simulink model "test"  (Simulink 6.4)
settings: Solver=FixedStepDiscrete  StartTime=0.0  StopTime=10.0  FixedStep=1  RelTol=1e-3
libraries: simulink x2
settings Model: Creator=brownm5  LastModifiedBy=brownm5
settings OptimizationCC: InlineInvariantSignals=on
settings DebuggingCC: StrictBusMsg=None
settings HardwareCC: TargetHWDeviceType=32-bit Generic

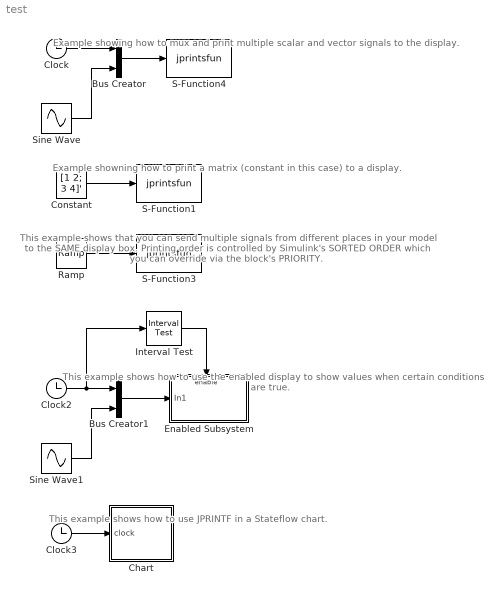
== system test ==
  note: Example showing how to mux and print multiple
      | scalar and vector signals to the display.
  note: Example showning how to print a matrix (constant
      | in this case) to a display.
  note: This example shows that you can send multiple
      | signals from different places in your model to
      | the SAME display box.  Printing order is controlled
      | by Simulink's SORTED ORDER which you can
      | override via the block's PRIORITY.
  note: This example shows how to use the enabled
      | display to show values when certain
      | conditions are true.
  note: This example shows how to use JPRINTF in a Stateflow chart.
  Bus Creator : BusCreator  Inputs=2
  Bus Creator1 : BusCreator  Inputs=2
  Chart : Stateflow chart  TreatAsAtomicUnit=on
      settings: PermitHierarchicalResolution=ParametersOnly
  Clock : Clock
      settings: Decimation=10
  Clock2 : Clock
      settings: Decimation=10
  Clock3 : Clock
      settings: Decimation=10
  Constant : Constant  Value=[1 2; 3 4]'  OutDataType=sfix(16)  OutScaling=2^0  SampleTime=1
  Enabled Subsystem : Subsystem  TreatAsAtomicUnit=on  mask(Java Display Box){dev=2, fmt1=Time\t\tSine 1\t\tSine 2\n, fmt2=, fmt3=%4.1f\t\t%6.3f\t\t%6.3f, fmt4=\n, fmt5=\nFinal values:\n, fmt6=%4.1f\t\t%6.3f\t\t%6.3f, fmt7=\n\n}
      mask prompts: dev "Display number"; fmt1 "Initialization format"; fmt2 "Update leader format"; fmt3 "Update numeric format"; fmt4 "Update trailer format"; fmt5 "Termination leader format"; fmt6 "Termination numeric format"; fmt7 "Termination trailer format"
      mask help:
      | Displays formatted text and numeric data to an editable Java window.
      | "Display Number" is a positive integer which specifies the Java window to receive the formatted output. Seven format strings control the appearance of the output during block initialization, update, and termination.  These strings can contain any combination of text and format specifiers acceptable to the Matlab FPRINTF function.
      |
      | See HELP for more information.
      mask Help:
      | <HTML>
      | 
      | <head>
      | <TITLE>Java Display Box</TITLE>
      | </head>
      | 
      | <body>
      | 
      | <h2>Function</h2>
      | Displays formatted text and numeric data to an editable Java window.
      | "Display Number" is a positive integer which specifies the Java window to receive the
      | formatted output. Seven format strings control the appearance of the output during
      | block initialization, update, and termination.  These strings can contain any combination
      | of text and format specifiers acceptable to the Matlab FPRINTF function.
      | 
      | <h2>Inputs</h2>
      | Java Display Box accepts any Simulink scalar, vector, or matrix signal.  The signal
      | must be real and double precision.  It is up to the user to perform data type conversion
      | (e.g. int8 to double) and to break apart complex signals into separate real and
      | imaginary parts.  This function will accept multiplexed signals and bus signals.  When
      | displaying matrix signals, Java Display Box will access the matrix data in columnwise
      | order, so you may need to transpose the matrix to display the matrix in it's natural
      | orientation.
      | 
      | <h2>Parameters</h2>
      | 
      | <h3>Display Number:</h3>
      | The display number is a numeric identifier for each active Java Display Box.  Any
      | positive integer greater than zero is acceptable.  If you want the outputs to go do
      | different windows, use differerent Display Numbers for each Java Display Box.
      | You can send multiple signals to the same window by using the same Display
      | Number.  In this case, the order in which the output is written to the box depends on
      | Simulink's execution order, called Sorted Order.  You can force multiple outputs to be
      | displayed in any desired sequence by overriding Simulink's Sorted Order using the
      | block priority property.  To change a Java Display Box priority, right-click the Java Box,
      | select Block  Properties, and enter a numeric value for Block Priority.  The lower the
      | number, the higher the priority, so a good rule of thumb is to assign priorities in the
      | order in which  you want the output to appear in the Java Display Box.
      | <br><br>
      | Note that multiple models share the same set of Java Display Boxes, so if you have
      | more than one model open and those models all access Display Box 1, then the
      | outputs from both models will appear in the same display window.
      | <br><br>
      | If you set the Display Number to -1, the outputs will go to the "standard output", normally
      | the Matlab command window.  A Display Number of -2 will send output to "standard
      | error", and a Display Number consisting of a valid handle to an open file will cause
      | the output to be written to the file.  The user is responsible for opening and closing
      | the file, and passing the file handle to Java Display Box.
      | 
      | <h3>Initialization Format:</h3>
      | The initialization format string is written once during model initialization.  Enter any valid
      | format string (without quotation marks!).  Note that during initialization, the input signal
      | values are generally undefined, so it is not possible to display numeric values of input
      | signals during initialization.  The Initialization Format is generally useful for printing
      | column headers or other delimiters to mark the beginning of a simulation run.  If you
      | don't want any initialization format, leave this field completely blank (i.e. no spaces or
      | other characters).
      | 
      | <h3>Update Format:</h3>
      | The update format strings consist of three parts:  Leader Format, Numeric Format, and
      | Trailer Format.  At each Simulink update time step, the Leader Format is first written
      | once.  Then the Numeric Format is applied to the input signal data, and repeated as
      | necessary to display all of the inputs.  Finally, the Trailer Format is written.  Typically,
      | the Leader Format contains textual information, such as 'Signal Amplitude = ', the
      | Numeric Format contains number formatting strings such as '%6.4f', and the Trailer
      | Format contains units and carriage controls such as '(volts)\n'.
      | 
      | <br><br>Be carefull!  If you have a lengthy simulation, or one that involves many time
      | steps, you can overrun the display memory.  If this is a possibility, consider using a
      | downsampler block in front of the Java Display Box, or enclose it in a triggered
      | subsystem so that only selected time samples are displayed.  If you don't want a
      | Leader, Numeric, or Trailer format, leave the field completely blank.
      | 
      | <h3>Termination Format:</h3>
      | The termination format string consists of three parts:  Leader Format, Numeric Format,
      | and Trailer Format.   These three formats are applied once at the end of a Simulink
      | simulation run.   First, the Leader Format is written once.  Then the Numeric Format is
      | applied to the input signal data, and repeated as necessary to display all of the inputs.
      | Finally, the Trailer Format is written.  Typically, the Leader Format contains textual
      | information, such as 'Signal Amplitude = ', the Numeric Format contains number
      | formatting strings such as '%6.4f', and the Trailer Format contains units and carriage
      | controls such as '(volts)\n'.  These formats are useful if you only want to display the
      | final values of signals at the end of simulation.  You can also use these fields to print
      | summary information, or model termination status.  If you don't want a Leader,
      | Numeric, or Trailer format, leave the field completely blank.
      | 
      | <h2>Java Display Box Menu:</h2>
      | These are fairly self-explanatory.  See HELP on the Java Box pulldown menu for more information.
      | 
      | </body>
      | 
      | </html>
      mask Display: fprintf('Enabled\nJava Box %d',dev)
  Interval Test : simulink/Logic and Bit Operations/Interval Test  SystemSampleTime=-1  IntervalClosedRight=on  uplimit=8  IntervalClosedLeft=on  lowlimit=5  LogicOutDataTypeMode=boolean
  Ramp : simulink/Sources/Ramp  SystemSampleTime=-1  slope=pi  start=0  X0=0
  S-Function1 : S-Function  Priority=4  FunctionName=jprintsfun  Parameters=dev,{fmt1,fmt2,fmt3,fmt4,fmt5,fmt6,fmt7}  EnableBusSupport=off  mask(Java Display Box){dev=1, fmt1=, fmt2=Matrix:\n, fmt3=\t%g\t%g\n, fmt4=\n, fmt5=, fmt6=, fmt7=}
      mask prompts: dev "Display number"; fmt1 "Initialization format"; fmt2 "Update leader format"; fmt3 "Update numeric format"; fmt4 "Update trailer format"; fmt5 "Termination leader format"; fmt6 "Termination numeric format"; fmt7 "Termination trailer format"
      mask help:
      | Displays formatted text and numeric data to an editable Java window.
      | "Display Number" is a positive integer which specifies the Java window to receive the formatted output. Seven format strings control the appearance of the output during block initialization, update, and termination.  These strings can contain any combination of text and format specifiers acceptable to the Matlab FPRINTF function.
      |
      | See HELP for more information.
      mask Help:
      | <HTML>
      | 
      | <head>
      | <TITLE>Java Display Box</TITLE>
      | </head>
      | 
      | <body>
      | 
      | <h2>Function</h2>
      | Displays formatted text and numeric data to an editable Java window.
      | "Display Number" is a positive integer which specifies the Java window to receive the
      | formatted output. Seven format strings control the appearance of the output during
      | block initialization, update, and termination.  These strings can contain any combination
      | of text and format specifiers acceptable to the Matlab FPRINTF function.
      | 
      | <h2>Inputs</h2>
      | Java Display Box accepts any Simulink scalar, vector, or matrix signal.  The signal
      | must be real and double precision.  It is up to the user to perform data type conversion
      | (e.g. int8 to double) and to break apart complex signals into separate real and
      | imaginary parts.  This function will accept multiplexed signals and bus signals.  When
      | displaying matrix signals, Java Display Box will access the matrix data in columnwise
      | order, so you may need to transpose the matrix to display the matrix in it's natural
      | orientation.
      | 
      | <h2>Parameters</h2>
      | 
      | <h3>Display Number:</h3>
      | The display number is a numeric identifier for each active Java Display Box.  Any
      | positive integer greater than zero is acceptable.  If you want the outputs to go do
      | different windows, use differerent Display Numbers for each Java Display Box.
      | You can send multiple signals to the same window by using the same Display
      | Number.  In this case, the order in which the output is written to the box depends on
      | Simulink's execution order, called Sorted Order.  You can force multiple outputs to be
      | displayed in any desired sequence by overriding Simulink's Sorted Order using the
      | block priority property.  To change a Java Display Box priority, right-click the Java Box,
      | select Block  Properties, and enter a numeric value for Block Priority.  The lower the
      | number, the higher the priority, so a good rule of thumb is to assign priorities in the
      | order in which  you want the output to appear in the Java Display Box.
      | <br><br>
      | Note that multiple models share the same set of Java Display Boxes, so if you have
      | more than one model open and those models all access Display Box 1, then the
      | outputs from both models will appear in the same display window.
      | <br><br>
      | If you set the Display Number to -1, the outputs will go to the "standard output", normally
      | the Matlab command window.  A Display Number of -2 will send output to "standard
      | error", and a Display Number consisting of a valid handle to an open file will cause
      | the output to be written to the file.  The user is responsible for opening and closing
      | the file, and passing the file handle to Java Display Box.
      | 
      | <h3>Initialization Format:</h3>
      | The initialization format string is written once during model initialization.  Enter any valid
      | format string (without quotation marks!).  Note that during initialization, the input signal
      | values are generally undefined, so it is not possible to display numeric values of input
      | signals during initialization.  The Initialization Format is generally useful for printing
      | column headers or other delimiters to mark the beginning of a simulation run.  If you
      | don't want any initialization format, leave this field completely blank (i.e. no spaces or
      | other characters).
      | 
      | <h3>Update Format:</h3>
      | The update format strings consist of three parts:  Leader Format, Numeric Format, and
      | Trailer Format.  At each Simulink update time step, the Leader Format is first written
      | once.  Then the Numeric Format is applied to the input signal data, and repeated as
      | necessary to display all of the inputs.  Finally, the Trailer Format is written.  Typically,
      | the Leader Format contains textual information, such as 'Signal Amplitude = ', the
      | Numeric Format contains number formatting strings such as '%6.4f', and the Trailer
      | Format contains units and carriage controls such as '(volts)\n'.
      | 
      | <br><br>Be carefull!  If you have a lengthy simulation, or one that involves many time
      | steps, you can overrun the display memory.  If this is a possibility, consider using a
      | downsampler block in front of the Java Display Box, or enclose it in a triggered
      | subsystem so that only selected time samples are displayed.  If you don't want a
      | Leader, Numeric, or Trailer format, leave the field completely blank.
      | 
      | <h3>Termination Format:</h3>
      | The termination format string consists of three parts:  Leader Format, Numeric Format,
      | and Trailer Format.   These three formats are applied once at the end of a Simulink
      | simulation run.   First, the Leader Format is written once.  Then the Numeric Format is
      | applied to the input signal data, and repeated as necessary to display all of the inputs.
      | Finally, the Trailer Format is written.  Typically, the Leader Format contains textual
      | information, such as 'Signal Amplitude = ', the Numeric Format contains number
      | formatting strings such as '%6.4f', and the Trailer Format contains units and carriage
      | controls such as '(volts)\n'.  These formats are useful if you only want to display the
      | final values of signals at the end of simulation.  You can also use these fields to print
      | summary information, or model termination status.  If you don't want a Leader,
      | Numeric, or Trailer format, leave the field completely blank.
      | 
      | <h2>Java Display Box Menu:</h2>
      | These are fairly self-explanatory.  See HELP on the Java Box pulldown menu for more information.
      | 
      | </body>
      | 
      | </html>
      mask Display: disp(['Java Box ',num2str(dev)])
  S-Function3 : S-Function  Priority=4  FunctionName=jprintsfun  Parameters=dev,{fmt1,fmt2,fmt3,fmt4,fmt5,fmt6,fmt7}  EnableBusSupport=off  mask(Java Display Box){dev=1, fmt1=, fmt2=Value of ramp =, fmt3=%g, fmt4=\n, fmt5=, fmt6=, fmt7=}
      mask prompts: dev "Display number"; fmt1 "Initialization format"; fmt2 "Update leader format"; fmt3 "Update numeric format"; fmt4 "Update trailer format"; fmt5 "Termination leader format"; fmt6 "Termination numeric format"; fmt7 "Termination trailer format"
      mask help:
      | Displays formatted text and numeric data to an editable Java window.
      | "Display Number" is a positive integer which specifies the Java window to receive the formatted output. Seven format strings control the appearance of the output during block initialization, update, and termination.  These strings can contain any combination of text and format specifiers acceptable to the Matlab FPRINTF function.
      |
      | See HELP for more information.
      mask Help:
      | <HTML>
      | 
      | <head>
      | <TITLE>Java Display Box</TITLE>
      | </head>
      | 
      | <body>
      | 
      | <h2>Function</h2>
      | Displays formatted text and numeric data to an editable Java window.
      | "Display Number" is a positive integer which specifies the Java window to receive the
      | formatted output. Seven format strings control the appearance of the output during
      | block initialization, update, and termination.  These strings can contain any combination
      | of text and format specifiers acceptable to the Matlab FPRINTF function.
      | 
      | <h2>Inputs</h2>
      | Java Display Box accepts any Simulink scalar, vector, or matrix signal.  The signal
      | must be real and double precision.  It is up to the user to perform data type conversion
      | (e.g. int8 to double) and to break apart complex signals into separate real and
      | imaginary parts.  This function will accept multiplexed signals and bus signals.  When
      | displaying matrix signals, Java Display Box will access the matrix data in columnwise
      | order, so you may need to transpose the matrix to display the matrix in it's natural
      | orientation.
      | 
      | <h2>Parameters</h2>
      | 
      | <h3>Display Number:</h3>
      | The display number is a numeric identifier for each active Java Display Box.  Any
      | positive integer greater than zero is acceptable.  If you want the outputs to go do
      | different windows, use differerent Display Numbers for each Java Display Box.
      | You can send multiple signals to the same window by using the same Display
      | Number.  In this case, the order in which the output is written to the box depends on
      | Simulink's execution order, called Sorted Order.  You can force multiple outputs to be
      | displayed in any desired sequence by overriding Simulink's Sorted Order using the
      | block priority property.  To change a Java Display Box priority, right-click the Java Box,
      | select Block  Properties, and enter a numeric value for Block Priority.  The lower the
      | number, the higher the priority, so a good rule of thumb is to assign priorities in the
      | order in which  you want the output to appear in the Java Display Box.
      | <br><br>
      | Note that multiple models share the same set of Java Display Boxes, so if you have
      | more than one model open and those models all access Display Box 1, then the
      | outputs from both models will appear in the same display window.
      | <br><br>
      | If you set the Display Number to -1, the outputs will go to the "standard output", normally
      | the Matlab command window.  A Display Number of -2 will send output to "standard
      | error", and a Display Number consisting of a valid handle to an open file will cause
      | the output to be written to the file.  The user is responsible for opening and closing
      | the file, and passing the file handle to Java Display Box.
      | 
      | <h3>Initialization Format:</h3>
      | The initialization format string is written once during model initialization.  Enter any valid
      | format string (without quotation marks!).  Note that during initialization, the input signal
      | values are generally undefined, so it is not possible to display numeric values of input
      | signals during initialization.  The Initialization Format is generally useful for printing
      | column headers or other delimiters to mark the beginning of a simulation run.  If you
      | don't want any initialization format, leave this field completely blank (i.e. no spaces or
      | other characters).
      | 
      | <h3>Update Format:</h3>
      | The update format strings consist of three parts:  Leader Format, Numeric Format, and
      | Trailer Format.  At each Simulink update time step, the Leader Format is first written
      | once.  Then the Numeric Format is applied to the input signal data, and repeated as
      | necessary to display all of the inputs.  Finally, the Trailer Format is written.  Typically,
      | the Leader Format contains textual information, such as 'Signal Amplitude = ', the
      | Numeric Format contains number formatting strings such as '%6.4f', and the Trailer
      | Format contains units and carriage controls such as '(volts)\n'.
      | 
      | <br><br>Be carefull!  If you have a lengthy simulation, or one that involves many time
      | steps, you can overrun the display memory.  If this is a possibility, consider using a
      | downsampler block in front of the Java Display Box, or enclose it in a triggered
      | subsystem so that only selected time samples are displayed.  If you don't want a
      | Leader, Numeric, or Trailer format, leave the field completely blank.
      | 
      | <h3>Termination Format:</h3>
      | The termination format string consists of three parts:  Leader Format, Numeric Format,
      | and Trailer Format.   These three formats are applied once at the end of a Simulink
      | simulation run.   First, the Leader Format is written once.  Then the Numeric Format is
      | applied to the input signal data, and repeated as necessary to display all of the inputs.
      | Finally, the Trailer Format is written.  Typically, the Leader Format contains textual
      | information, such as 'Signal Amplitude = ', the Numeric Format contains number
      | formatting strings such as '%6.4f', and the Trailer Format contains units and carriage
      | controls such as '(volts)\n'.  These formats are useful if you only want to display the
      | final values of signals at the end of simulation.  You can also use these fields to print
      | summary information, or model termination status.  If you don't want a Leader,
      | Numeric, or Trailer format, leave the field completely blank.
      | 
      | <h2>Java Display Box Menu:</h2>
      | These are fairly self-explanatory.  See HELP on the Java Box pulldown menu for more information.
      | 
      | </body>
      | 
      | </html>
      mask Display: disp(['Java Box ',num2str(dev)])
  S-Function4 : S-Function  Priority=4  FunctionName=jprintsfun  Parameters=dev,{fmt1,fmt2,fmt3,fmt4,fmt5,fmt6,fmt7}  EnableBusSupport=off  mask(Java Display Box){dev=4, fmt1=Time\t\tSine 1\t\tSine 2\n, fmt2=, fmt3=%4.1f\t\t%6.3f\t\t%6.3f, fmt4=\n, fmt5=\nFinal values:\n, fmt6=%4.1f\t\t%6.3f\t\t%6.3f, fmt7=\n}
      mask prompts: dev "Display number"; fmt1 "Initialization format"; fmt2 "Update leader format"; fmt3 "Update numeric format"; fmt4 "Update trailer format"; fmt5 "Termination leader format"; fmt6 "Termination numeric format"; fmt7 "Termination trailer format"
      mask help:
      | Displays formatted text and numeric data to an editable Java window.
      | "Display Number" is a positive integer which specifies the Java window to receive the formatted output. Seven format strings control the appearance of the output during block initialization, update, and termination.  These strings can contain any combination of text and format specifiers acceptable to the Matlab FPRINTF function.
      |
      | See HELP for more information.
      mask Help:
      | <HTML>
      | 
      | <head>
      | <TITLE>Java Display Box</TITLE>
      | </head>
      | 
      | <body>
      | 
      | <h2>Function</h2>
      | Displays formatted text and numeric data to an editable Java window.
      | "Display Number" is a positive integer which specifies the Java window to receive the
      | formatted output. Seven format strings control the appearance of the output during
      | block initialization, update, and termination.  These strings can contain any combination
      | of text and format specifiers acceptable to the Matlab FPRINTF function.
      | 
      | <h2>Inputs</h2>
      | Java Display Box accepts any Simulink scalar, vector, or matrix signal.  The signal
      | must be real and double precision.  It is up to the user to perform data type conversion
      | (e.g. int8 to double) and to break apart complex signals into separate real and
      | imaginary parts.  This function will accept multiplexed signals and bus signals.  When
      | displaying matrix signals, Java Display Box will access the matrix data in columnwise
      | order, so you may need to transpose the matrix to display the matrix in it's natural
      | orientation.
      | 
      | <h2>Parameters</h2>
      | 
      | <h3>Display Number:</h3>
      | The display number is a numeric identifier for each active Java Display Box.  Any
      | positive integer greater than zero is acceptable.  If you want the outputs to go do
      | different windows, use differerent Display Numbers for each Java Display Box.
      | You can send multiple signals to the same window by using the same Display
      | Number.  In this case, the order in which the output is written to the box depends on
      | Simulink's execution order, called Sorted Order.  You can force multiple outputs to be
      | displayed in any desired sequence by overriding Simulink's Sorted Order using the
      | block priority property.  To change a Java Display Box priority, right-click the Java Box,
      | select Block  Properties, and enter a numeric value for Block Priority.  The lower the
      | number, the higher the priority, so a good rule of thumb is to assign priorities in the
      | order in which  you want the output to appear in the Java Display Box.
      | <br><br>
      | Note that multiple models share the same set of Java Display Boxes, so if you have
      | more than one model open and those models all access Display Box 1, then the
      | outputs from both models will appear in the same display window.
      | <br><br>
      | If you set the Display Number to -1, the outputs will go to the "standard output", normally
      | the Matlab command window.  A Display Number of -2 will send output to "standard
      | error", and a Display Number consisting of a valid handle to an open file will cause
      | the output to be written to the file.  The user is responsible for opening and closing
      | the file, and passing the file handle to Java Display Box.
      | 
      | <h3>Initialization Format:</h3>
      | The initialization format string is written once during model initialization.  Enter any valid
      | format string (without quotation marks!).  Note that during initialization, the input signal
      | values are generally undefined, so it is not possible to display numeric values of input
      | signals during initialization.  The Initialization Format is generally useful for printing
      | column headers or other delimiters to mark the beginning of a simulation run.  If you
      | don't want any initialization format, leave this field completely blank (i.e. no spaces or
      | other characters).
      | 
      | <h3>Update Format:</h3>
      | The update format strings consist of three parts:  Leader Format, Numeric Format, and
      | Trailer Format.  At each Simulink update time step, the Leader Format is first written
      | once.  Then the Numeric Format is applied to the input signal data, and repeated as
      | necessary to display all of the inputs.  Finally, the Trailer Format is written.  Typically,
      | the Leader Format contains textual information, such as 'Signal Amplitude = ', the
      | Numeric Format contains number formatting strings such as '%6.4f', and the Trailer
      | Format contains units and carriage controls such as '(volts)\n'.
      | 
      | <br><br>Be carefull!  If you have a lengthy simulation, or one that involves many time
      | steps, you can overrun the display memory.  If this is a possibility, consider using a
      | downsampler block in front of the Java Display Box, or enclose it in a triggered
      | subsystem so that only selected time samples are displayed.  If you don't want a
      | Leader, Numeric, or Trailer format, leave the field completely blank.
      | 
      | <h3>Termination Format:</h3>
      | The termination format string consists of three parts:  Leader Format, Numeric Format,
      | and Trailer Format.   These three formats are applied once at the end of a Simulink
      | simulation run.   First, the Leader Format is written once.  Then the Numeric Format is
      | applied to the input signal data, and repeated as necessary to display all of the inputs.
      | Finally, the Trailer Format is written.  Typically, the Leader Format contains textual
      | information, such as 'Signal Amplitude = ', the Numeric Format contains number
      | formatting strings such as '%6.4f', and the Trailer Format contains units and carriage
      | controls such as '(volts)\n'.  These formats are useful if you only want to display the
      | final values of signals at the end of simulation.  You can also use these fields to print
      | summary information, or model termination status.  If you don't want a Leader,
      | Numeric, or Trailer format, leave the field completely blank.
      | 
      | <h2>Java Display Box Menu:</h2>
      | These are fairly self-explanatory.  See HELP on the Java Box pulldown menu for more information.
      | 
      | </body>
      | 
      | </html>
      mask Display: disp(['Java Box ',num2str(dev)])
  Sine Wave : Sin  Amplitude=[1 2]  Bias=0  Frequency=1  Phase=[0 pi/3]  Samples=10  SampleTime=0  Offset=0
  Sine Wave1 : Sin  Amplitude=[1 2]  Bias=0  Frequency=1  Phase=[0 pi/3]  Samples=10  SampleTime=0  Offset=0
  wires:
  Sine Wave/1 -> Bus Creator/2
  Clock/1 -> Bus Creator/1
  Bus Creator/1 -> S-Function4/1
  Constant/1 -> S-Function1/1
  Interval Test/1 -> Enabled Subsystem/Enable
  Clock3/1 -> Chart/1(clock)
  Sine Wave1/1 -> Bus Creator1/2
  Clock2/1 -> Bus Creator1/1, Interval Test/1
  Bus Creator1/1 -> Enabled Subsystem/1(In1)
  Ramp/1 -> S-Function3/1

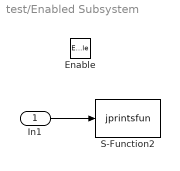
== system test/Enabled Subsystem ==
  In1 : Inport  OutDataType=sfix(16)  OutScaling=2^0
  Enable : EnablePort
  S-Function2 : S-Function  Priority=4  FunctionName=jprintsfun  Parameters=dev,{fmt1,fmt2,fmt3,fmt4,fmt5,fmt6,fmt7}  EnableBusSupport=off
  wires:
  In1/1 -> S-Function2/1

== stateflow chart Chart ==
  settings: updateMethod=DISCRETE  sampleTime=1
  state Anystate
    entry: y = x*3;
    ml.jprintf(-3,'This was printed from within a STATE\n');
    disp(clock,x,y);
  state disp(t,xin,yin) [function]
    (default) -> (junction 8) : {ml.jprintf(-3,'Stateflow Time=%6.4f\n',t);
        | ml.jprintf(-3,'Data Values:\tX=%g,\tY = %g\n',xin,yin);}
  note: This chart is set up for a fixed update
      | rate of 1.0 and to automatically enter the
      | chart at startup.
  note: Variables x and y are local.  An external
      | clock is input from Simulink to show how
      | to display event time.
  note: Note when calling JPRINTF directly,
      | you must use a NEGATIVE device
      | specifier -- unlike the Java Box in
      | Simulink (which adds the minus sign
      | for you).
  (default) -> Anystate : {x=1.234;}
  data: t function_input double; xin function_input double; yin function_input double; x local double; y local double; clock input double
